simulink model "Project_Part2"  (R2021a)
settings: Solver=VariableStepAuto  StartTime=0.0  StopTime=Time_stop  MaxStep=1e-3  RelTol=1e-3
values from neighbouring files (symbols this model uses):
  g = 9.81    [Project_Script_Part2.m]
  L = values_Of_L(i)    [Project_Script_Part2.m]
  theta_0 = 40    [Project_Script_Part2.m]
settings Model: Creator=MAC  LastModifiedBy=MAC

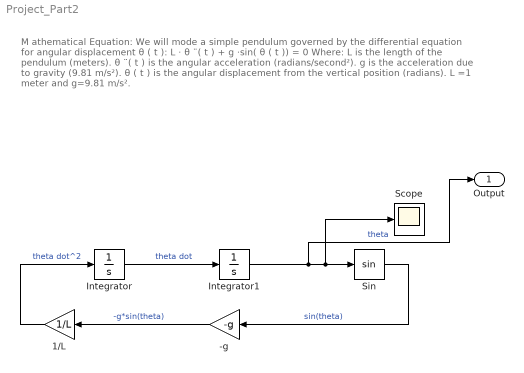
== system Project_Part2 ==
  note: M athematical Equation:
      | We will mode a simple pendulum governed by the differential equation for angular displacement θ ( t ):
      | L ⋅ θ ¨( t ) + g ⋅sin( θ ( t )) = 0
      | Where:
      | L is the length of the pendulum (meters).
      | θ ¨( t ) is the angular acceleration (radians/second²).
      | g is the acceleration due to gravity (9.81 m/s²).
      | θ ( t ) is the angular displacement from the vertical position (radians).
      | L =1 meter and g=9.81 m/s².
  -g : Gain  Gain=-g
  1/L : Gain  Gain=1/L
  Integrator : Integrator
  Integrator1 : Integrator  InitialCondition=theta_0
  Scope : Scope
  Sin : Trigonometry
  Output : Outport
  wires:
  Integrator1/1 -> Output/1, Scope/1, Sin/1  "theta"
  Sin/1 -> -g/1  "sin(theta)"
  -g/1 -> 1/L/1  "-g*sin(theta)"
  Integrator/1 -> Integrator1/1  "theta dot"
  1/L/1 -> Integrator/1  "theta dot^2"
